simulink model "slip_ground_memoria"  (R2019a)
settings: Solver=VariableStepAuto  StartTime=0.0  StopTime=tc  RelTol=1e-1
values from neighbouring files (symbols this model uses):
  g = -9.81    [SLIP.m]    (also in SLIP_alfa0.m; slipFarley93.m)
  k = 2000.0    (= 2000)    [SLIP.m]    (also in SLIP_alfa0.m = 22500; slipFarley93.m = 4960)
  L0 = Lhk + Lkf    (= 0.56)    [SLIP.m]    (also in SLIP_alfa0.m; slipFarley93.m)
  Lcol = 0.70    (= 0.7)    [SLIP.m]
  Lhk = 0.28    [SLIP.m]
  Lkf = 0.28    [SLIP.m]
  M = 15+3    (= 18)    [SLIP.m]    (also in SLIP_alfa0.m; slipFarley93.m)
  vx0 = vxairSlip( length(vxairSlip) )    [SLIP.m]    (also in SLIP_alfa0.m = 0; slipFarley93.m = 0)
  vy0 = vyairSlip( length(vyairSlip) )    [SLIP.m]    (also in SLIP_alfa0.m = -0.7; slipFarley93.m = -0.7)
  x0 = L0 * sin(alfa0)    [SLIP.m]    (also in SLIP_alfa0.m = 0; slipFarley93.m)
  y0 = L0 * cos(alfa0)    [SLIP.m]    (also in SLIP_alfa0.m = 0.56; slipFarley93.m)
undefined symbols (not defined in the file or in its folder): magnitude
settings Model: Creator=Jesus  LastModifiedBy=Jesus

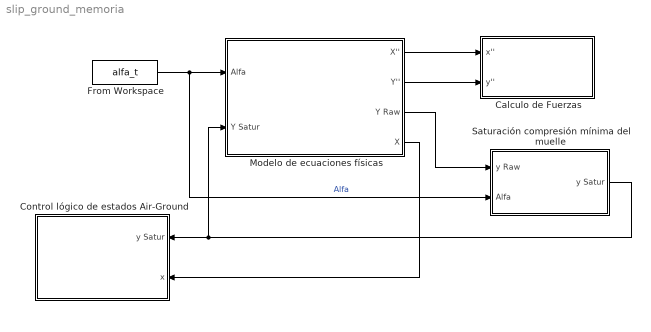
== system slip_ground_memoria ==
  Calculo de Fuerzas : Subsystem
  Control lógico de estados Air-Ground : Subsystem
  From Workspace : FromWorkspace  VariableName=alfa_t  SampleTime=0
  Modelo de ecuaciones físicas : Subsystem
  Saturación compresión mínima del muelle : Subsystem
  wires:
  From Workspace/1 -> Saturación compresión mínima del muelle/2(Alfa), Modelo de ecuaciones físicas/1(Alfa)  "Alfa"
  Saturación compresión mínima del muelle/1(y Satur) -> Modelo de ecuaciones físicas/2(Y Satur), Control lógico de estados Air-Ground/1(y Satur)
  Modelo de ecuaciones físicas/3(Y Raw) -> Saturación compresión mínima del muelle/1(y Raw)
  Modelo de ecuaciones físicas/1(X'') -> Calculo de Fuerzas/1(x'')
  Modelo de ecuaciones físicas/2(Y'') -> Calculo de Fuerzas/2(y'')
  Modelo de ecuaciones físicas/4(X) -> Control lógico de estados Air-Ground/2(x)

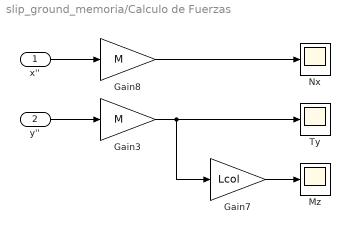
== system slip_ground_memoria/Calculo de Fuerzas ==
  x'' : Inport
  y'' : Inport  Port=2
  Gain3 : Gain  Gain=M
  Gain7 : Gain  Gain=Lcol
  Gain8 : Gain  Gain=M
  Mz : Scope
  Nx : Scope
  Ty : Scope
  wires:
  Gain8/1 -> Nx/1
  x''/1 -> Gain8/1
  Gain7/1 -> Mz/1
  y''/1 -> Gain3/1
  Gain3/1 -> Ty/1, Gain7/1

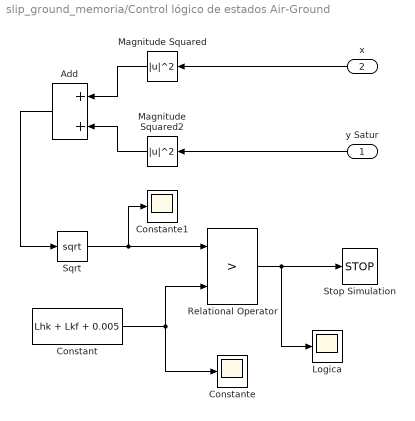
== system slip_ground_memoria/Control lógico de estados Air-Ground ==
  y Satur : Inport
  x : Inport  Port=2
  Add : Sum
  Constant : Constant  Value=Lhk + Lkf + 0.005
  Constante : Scope
  Constante1 : Scope
  Logica : Scope
  Magnitude Squared : Math  Operator=magnitude^2  SaturateOnIntegerOverflow=on
  Magnitude Squared2 : Math  Operator=magnitude^2  SaturateOnIntegerOverflow=on
  Relational Operator : RelationalOperator  Operator=>  OutDataTypeStr=boolean  RndMeth=Simplest
  Sqrt : Sqrt  SaturateOnIntegerOverflow=on
  Stop Simulation : Stop
  wires:
  Relational Operator/1 -> Logica/1, Stop Simulation/1
  Constant/1 -> Constante/1, Relational Operator/2
  Add/1 -> Sqrt/1
  Sqrt/1 -> Constante1/1, Relational Operator/1
  Magnitude Squared/1 -> Add/1
  y Satur/1 -> Magnitude Squared2/1
  x/1 -> Magnitude Squared/1
  Magnitude Squared2/1 -> Add/2

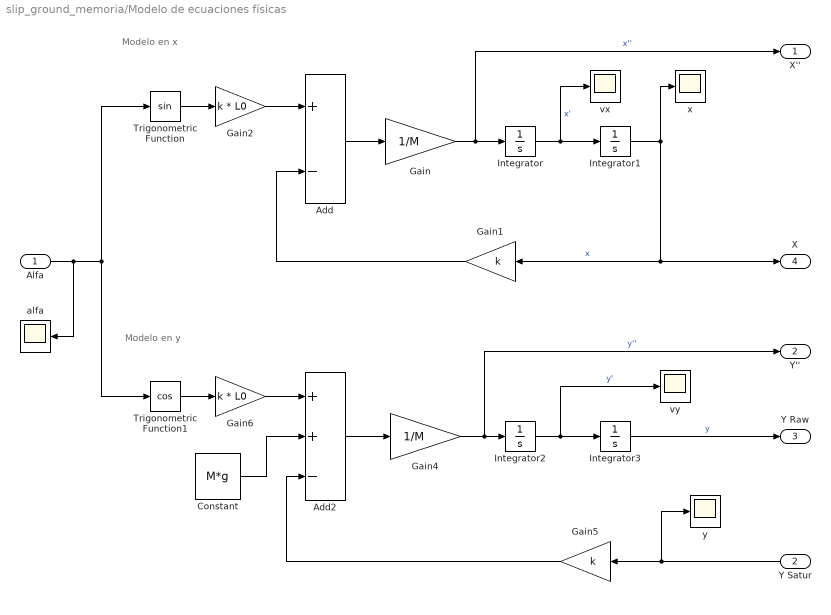
== system slip_ground_memoria/Modelo de ecuaciones físicas ==
  note: Modelo en x
  note: Modelo en y
  Alfa : Inport
  Y Satur : Inport  Port=2
  Add : Sum  Inputs=+-
  Add2 : Sum  Inputs=++-
  Constant : Constant  Value=M*g
  Gain : Gain  Gain=1/M
  Gain1 : Gain  Gain=k
  Gain2 : Gain  Gain=k * L0
  Gain4 : Gain  Gain=1/M
  Gain5 : Gain  Gain=k
  Gain6 : Gain  Gain=k * L0
  Integrator : Integrator  InitialCondition=vx0
  Integrator1 : Integrator  InitialCondition=x0
  Integrator2 : Integrator  InitialCondition=vy0
  Integrator3 : Integrator  InitialCondition=y0
  Trigonometric Function : Trigonometry
  Trigonometric Function1 : Trigonometry  Operator=cos
  alfa : Scope
  vx : Scope
  vy : Scope
  x : Scope
  y : Scope
  X'' : Outport
  Y'' : Outport  Port=2
  Y Raw : Outport  Port=3
  X : Outport  Port=4
  wires:
  Gain5/1 -> Add2/3
  Gain6/1 -> Add2/1
  Integrator/1 -> vx/1, Integrator1/1  "x'"
  Constant/1 -> Add2/2
  Integrator1/1 -> X/1, Gain1/1, x/1  "x"
  Integrator2/1 -> vy/1, Integrator3/1  "y'"
  Gain/1 -> X''/1, Integrator/1  "x''"
  Add2/1 -> Gain4/1
  Alfa/1 -> Trigonometric Function1/1, Trigonometric Function/1, alfa/1
  Trigonometric Function/1 -> Gain2/1
  Gain2/1 -> Add/1
  Gain4/1 -> Y''/1, Integrator2/1  "y''"
  Add/1 -> Gain/1
  Trigonometric Function1/1 -> Gain6/1
  Integrator3/1 -> Y Raw/1  "y"
  Gain1/1 -> Add/2
  Y Satur/1 -> y/1, Gain5/1

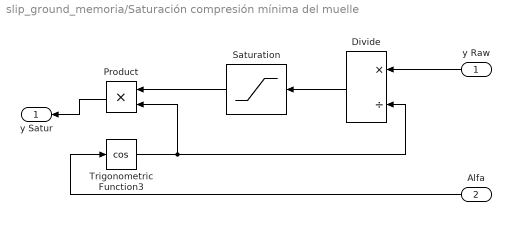
== system slip_ground_memoria/Saturación compresión mínima del muelle ==
  y Raw : Inport
  Alfa : Inport  Port=2
  Divide : Product  Inputs=*/
  Product : Product
  Saturation : Saturate  UpperLimit=inf  LowerLimit=-inf
  Trigonometric Function3 : Trigonometry  Operator=cos
  y Satur : Outport
  wires:
  Trigonometric Function3/1 -> Product/2, Divide/2
  Alfa/1 -> Trigonometric Function3/1
  y Raw/1 -> Divide/1
  Divide/1 -> Saturation/1
  Product/1 -> y Satur/1
  Saturation/1 -> Product/1
